simulink model "compareFlexibleCylinders"  (R2023a)
settings: Solver=ode23t  StartTime=0.0  StopTime=2.5  MaxStep=0.01  RelTol=1e-4  AbsTol=1e-5  EnableMultiTasking=on
PreLoadFcn:
  | setup_ROM_validation;
StopFcn:
  | show_SDI_view(ValidationTest)
undefined symbols (not defined in the file): E, L, nu, r, X, Y, Z
libraries: sm_lib x15, nesl_utility x7
settings Model: Creator=dbalbuen  LastModifiedBy=upattacini
settings SolverCC: AutoScaleAbsTol=off  AlgebraicLoopSolver=TrustRegion
settings DataIOCC: MaxDataPoints=10000  SaveOutput=off  DSMLogging=off  SignalLoggingName=logsout_flex_body  DatasetSignalFormat=timetable
settings OptimizationCC: ReuseModelBlockBuffer=off  LifeSpan=inf
settings DebuggingCC: UnconnectedInputMsg=warning  UnconnectedOutputMsg=warning  UnconnectedLineMsg=warning  AllowSymbolicDim=off  SFUnexpectedBacktrackingDiag=warning  SFNoUnconditionalDefaultTransitionDiag=warning  SFExecutionAtInitializationDiag=none  ArithmeticOperatorsInVariantConditions=warning
settings ModelReferenceCC: EnableRefExpFcnMdlSchedulingChecks=on
settings SFSimCC: SimUseLocalCustomCode=off  CustomCodeUndefinedFunction=UseInterfaceOnly
settings RTWCC: RTWUseLocalCustomCode=off  DLArmComputeVersion=19.05
settings CodeAppCC: StateflowObjectComments=on
settings GRTTargetCC: TargetLangStandard=C89/C90 (ANSI)
settings ConfigComp: CovMetricSettings=dw  CovSaveCumulativeToWorkspaceVar=on  CovSaveSingleToWorkspaceVar=on  CovExternalEMLEnable=off  CovSFcnEnable=off
settings SimscapeCC: SimscapeLogType=all  SimscapeLogSimulationStatistics=on  SimscapeLogDataHistory=10000
settings DiagnosticsConfigSet: SimMechanicsInvalidVisualProperty=none
settings ExplorerConfigSet: InternalSimMechanicsExplorerSettings="<ExplorerConfiguration><canonicalview>default</canonicalview><AnimationSetting><BasePlaybackSpeed>1.0</BasePlaybackSpeed><PlaybackSpeedFactor>1.0</PlaybackSpeedFactor></AnimationSetting><TilePanel><TileInfo><Tiles Columns=\"2\" Count=\"2\" Rows=\"1\"><Column Weight=\"0.4996\"/><Column Weight=\"0.5004\"/><Row Weight=\"1\"/><Tile Height=\"1\" Width=\"1\" X=\"0\" Y=\"0\"/><Tile Height=\"1\" Width=\"1\" X=\"1\" Y=\"0\"/></Tiles></TileInfo><SceneInfo><SceneViewer><BGColor><R>1</R><G>1</G><B>1</B></BGColor><Camera><DoPerspective>off</DoPerspective><Position><X>1.10451667165203782</X><Y>-0.556333933861863805</Y><Z>0.510096200126537114</Z></Position><Center><X>0.388367773315445863</X><Y>0.1598149644747279</Y><Z>-0.20605269821005473</Z></Center><Up><X>-0.408248290463863073</X><Y>0.408248290463863073</Y><Z>0.816496580927726145</Z></Up><ViewLimDist>1</ViewLimDist><YLim>0.805305415050960982</YLim><XLim>0.516336295324746897</XLim></Camera></SceneViewer><SceneViewer><BGColor><R>1</R><G>1</G><B>1</B></BGColor><Camera><DoPerspective>off</DoPerspective><Position><X>0.524478029771406673</X><Y>-1.08935703501999259</Y><Z>-0.311817888307719004</Z></Position><Center><X>0.524478029771406673</X><Y>1.33809996694100874e-08</Y><Z>-0.311817888307719004</Z></Center><Up><X>0</X><Y>-0</Y><Z>1</Z></Up><ViewLimDist>1</ViewLimDist><YLim>1.0281975000000001</YLim><XLim>0.660677670375521608</XLim></Camera></SceneViewer></SceneInfo></TilePanel><MechEditorPanel><Cameras/><GfxPanelCameraMap/><VideoCreator><PlaybackSpeedRatio>1.0</PlaybackSpeedRatio><FrameRate>30</FrameRate><VideoFormat>Motion JPEG AVI</VideoFormat><FrameSize>auto</FrameSize></VideoCreator></MechEditorPanel></ExplorerConfiguration>"

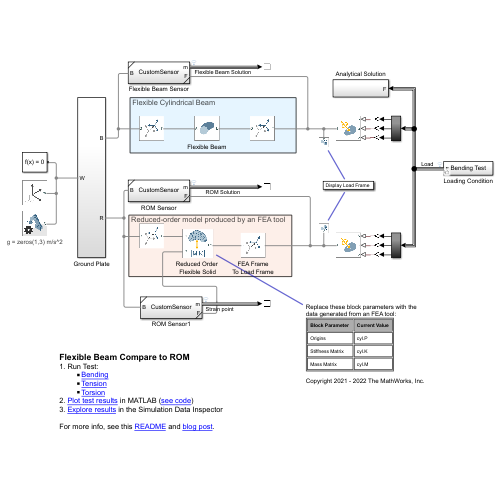
[thumbnail: Simulink's stored preview of the top-level diagram]
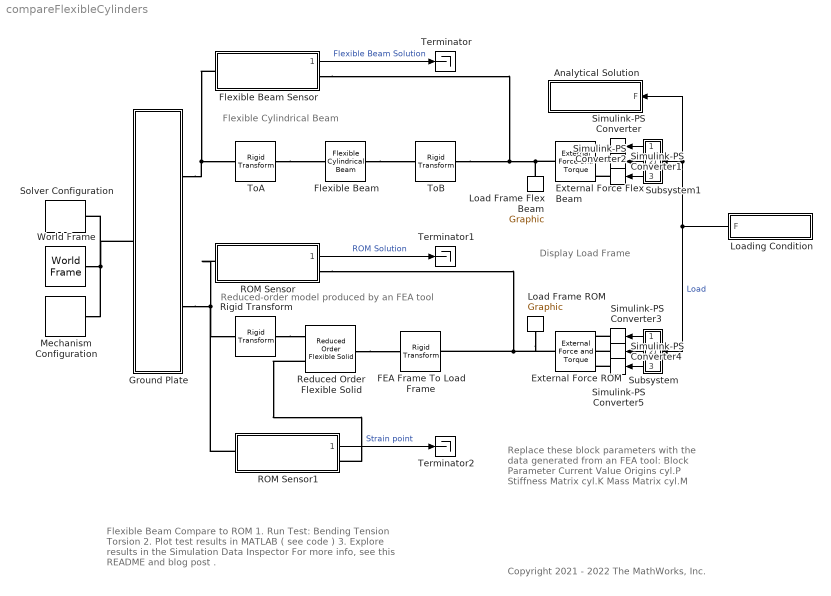
== system compareFlexibleCylinders ==
  note: Display Load Frame
  note: Replace these block parameters with the data generated from an FEA tool:
      |
      | Block Parameter
      | Current Value
      |
      | Origins
      | cyl.P
      |
      | Stiffness Matrix
      | cyl.K
      |
      | Mass Matrix
      | cyl.M
  note: Flexible Cylindrical Beam
  note: Reduced-order model produced by an FEA tool
  note: Flexible Beam Compare to ROM
      | 1. Run Test:
      | Bending
      | Tension
      | Torsion
      | 2. Plot test results in MATLAB ( see code )
      | 3. Explore results in the Simulation Data Inspector
      |
      | For more info, see this README and blog post .
  note: Copyright 2021 - 2022 The MathWorks, Inc.
  Analytical Solution : Subsystem
  External Force Flex Beam : sm_lib/Forces and Torques/External Force and Torque  ForceResolutionFrame=AttachedFrame  EnableForceX=on  EnableForceY=off  EnableForceZ=on  EnableForce=off  TorqueResolutionFrame=AttachedFrame  EnableTorqueX=on  EnableTorqueY=off  EnableTorqueZ=off  EnableTorque=off
  External Force ROM : sm_lib/Forces and Torques/External Force and Torque  ForceResolutionFrame=AttachedFrame  EnableForceX=on  EnableForceY=off  EnableForceZ=on  EnableForce=off  TorqueResolutionFrame=AttachedFrame  EnableTorqueX=on  EnableTorqueY=off  EnableTorqueZ=off  EnableTorque=off
  FEA Frame To Load Frame : sm_lib/Frames and Transforms/Rigid Transform  TranslationMethod=None  TranslationStandardOffset=0  TranslationStandardOffsetUnits=m  TranslationStandardAxis=+Z  TranslationCartesianOffset=[0 0 0]  TranslationCartesianOffsetUnits=m  TranslationROffset=0  TranslationROffsetUnits=m  TranslationZOffset=0  TranslationZOffsetUnits=m  TranslationThetaOffset=0  TranslationThetaOffsetUnits=deg  RotationMethod=StandardAxis  RotationAngleUnits=deg  RotationStandardAxis=+Y  RotationAngle=90  RotationArbitraryAxis=[0 0 1]  FollAlignAxisA=+X  BaseAlignAxisA=+Y  FollAlignAxisB=+Y  BaseAlignAxisB=+Z  RotationSequenceAxes=FollowerAxes  RotationSequence=XYX  RotationSequenceAngles=[0 0 0]  RotationSequenceAnglesUnits=deg  RotationMatrix=[1 0 0; 0 1 0; 0 0 1]  Quaternion=[1 0 0 0]
  Flexible Beam : sm_lib/Body Elements/Flexible Bodies/Beams/Flexible Cylindrical Beam  GraphicAmbientColor=[0.15 0.15 0.15 1.0]  AxialRigidity=1  AxialRigidityUnits=Pa*m^2  BendingCentroid=[0 0]  BendingCentroidUnits=m  FlexuralRigidity=[1 1]  FlexuralRigidityUnits=Pa*m^4  CenterOfMass=[0 0]  CenterOfMassUnits=m  GraphicDiffuseColor=[0.0 0.8 1.0]  CrossFlexuralRigidity=0  CrossFlexuralRigidityUnits=Pa*m^4  SerializedFrames=<Frames/>  DampingType=Proportional  Density=rho  DensityUnits=kg/m^3  DoExposeZmaxFrame=on  DoExposeZminFrame=on  GraphicEmissiveColor=[0.0 0.0 0.0 1.0]  GeometricCentroid=[0 0]  GeometricCentroidUnits=m  GraphicType=FromGeometry  Length=L  LengthUnits=m  MassMomentOfInertiaDensity=[1 1]  MassMomentOfInertiaDensityUnits=kg*m  MassPerUnitLength=1  MassPerUnitLengthUnits=kg/m  MassProductOfInertiaDensity=0  MassProductOfInertiaDensityUnits=kg*m  ModuliType=YoungsPoissons  NumElements=10  NumRetainedModes=1  GraphicOpacity=1  PoissonsRatio=nu  Radius=r  RadiusUnits=m  ReductionType=None  SectionType=Solid  ShearCenter=[0 0]  ShearCenterUnits=m  ShearModulus=26  ShearModulusUnits=GPa  GraphicShininess=75  GraphicSpecularColor=[0.5 0.5 0.5 1.0]  StiffnessAndInertiaType=CalculateFromGeometry  Thickness=0.1  ThicknessUnits=m  TorsionalRigidity=1  TorsionalRigidityUnits=Pa*m^4  GraphicVisPropType=SimpleVisualProperties  YoungsModulus=E  YoungsModulusUnits=Pa  ProportionalDampingAlpha=0  ProportionalDampingAlphaUnits=1/s  ProportionalDampingBeta=Beta  ProportionalDampingBetaUnits=s  UniformModalDampingRatio=0.01
  Flexible Beam Sensor : Subsystem  ReferencedSubsystem=CustomSensor
      settings: PortSchema="{\"entries\":[{\"content\":{\"sides\":[{\"content\":{\"connectorIds\":[\"LConn1\"]},\"type\":\"ConnectorPlacement.EquallySpacedRectSide\",\"uuid\":\"7fafd3ae-1fba-4f09-a97b-f3b2342423e3\"},{\"content\":{\"connectorIds\":[\"RConn1\",\"Out1\"],\"side\":\"RIGHT\"},\"type\":\"ConnectorPlacement.EquallySpacedRectSide\",\"uuid\":\"bc0d00af-c2a5-4688-9bba-52926bbc70a8\"},{\"content\":{\"side\":\"TOP\"},\"type\":\"ConnectorPlacement.EquallySpacedRectSide\",\"uuid\":\"984d0ed5-678d-4848-ae86-c23030322328\"},{\"content\":{\"side\":\"HIDDEN\"},\"type\":\"ConnectorPlacement.EquallySpacedRectSide\",\"uuid\":\"5459c863-0a9c-435c-a481-400fa9a25bf2\"}]},\"type\":\"ConnectorPlacement.EquallySpacedConnector\",\"uuid\":\"ae2cbc6a-d804-41f6-859e-ee34f76c879c\"}],\"packageUris\":[\"http://schema.mathworks.com/mf0/Connector/R2020b\"],\"version\":\"1.0\"}"
  Ground Plate : Subsystem
  Load Frame Flex Beam : sm_lib/Body Elements/Graphic  GraphicType=Marker  MarkerShape=Frame  MarkerSize=30  GraphicVisPropType=SimpleVisualProperties  GraphicDiffuseColor=[0.0 0.0 0.0]  GraphicSpecularColor=[0.5 0.5 0.5 1.0]  GraphicAmbientColor=[0.15 0.15 0.15 1.0]  GraphicEmissiveColor=[0.0 0.0 0.0 1.0]  GraphicShininess=75  GraphicOpacity=1.0
  Load Frame ROM : sm_lib/Body Elements/Graphic  GraphicType=Marker  MarkerShape=Frame  MarkerSize=30  GraphicVisPropType=SimpleVisualProperties  GraphicDiffuseColor=[0.0 0.0 0.0]  GraphicSpecularColor=[0.5 0.5 0.5 1.0]  GraphicAmbientColor=[0.15 0.15 0.15 1.0]  GraphicEmissiveColor=[0.0 0.0 0.0 1.0]  GraphicShininess=75  GraphicOpacity=1.0
  Loading Condition : Subsystem  Variant=on  VariantControl=Choice
  Mechanism Configuration : sm_lib/Utilities/Mechanism Configuration  UniformGravity=Constant  GravityVector=zeros(1,3)  GravityVectorUnits=m/s^2  LinearizationDelta=0.001  JointModeTransitionNonlinearIterations=2
      settings: AttributesFormatString=g = %<GravityVector> %<GravityVectorUnits>
  ROM Sensor : Subsystem  ReferencedSubsystem=CustomSensor
      settings: PortSchema="{\"entries\":[{\"content\":{\"sides\":[{\"content\":{\"connectorIds\":[\"LConn1\"]},\"type\":\"ConnectorPlacement.EquallySpacedRectSide\",\"uuid\":\"7fafd3ae-1fba-4f09-a97b-f3b2342423e3\"},{\"content\":{\"connectorIds\":[\"RConn1\",\"Out1\"],\"side\":\"RIGHT\"},\"type\":\"ConnectorPlacement.EquallySpacedRectSide\",\"uuid\":\"bc0d00af-c2a5-4688-9bba-52926bbc70a8\"},{\"content\":{\"side\":\"TOP\"},\"type\":\"ConnectorPlacement.EquallySpacedRectSide\",\"uuid\":\"984d0ed5-678d-4848-ae86-c23030322328\"},{\"content\":{\"side\":\"HIDDEN\"},\"type\":\"ConnectorPlacement.EquallySpacedRectSide\",\"uuid\":\"5459c863-0a9c-435c-a481-400fa9a25bf2\"}]},\"type\":\"ConnectorPlacement.EquallySpacedConnector\",\"uuid\":\"ae2cbc6a-d804-41f6-859e-ee34f76c879c\"}],\"packageUris\":[\"http://schema.mathworks.com/mf0/Connector/R2020b\"],\"version\":\"1.0\"}"
  ROM Sensor1 : Subsystem  ReferencedSubsystem=CustomSensor
      settings: PortSchema="{\"entries\":[{\"content\":{\"sides\":[{\"content\":{\"connectorIds\":[\"LConn1\"]},\"type\":\"ConnectorPlacement.EquallySpacedRectSide\",\"uuid\":\"7fafd3ae-1fba-4f09-a97b-f3b2342423e3\"},{\"content\":{\"connectorIds\":[\"RConn1\",\"Out1\"],\"side\":\"RIGHT\"},\"type\":\"ConnectorPlacement.EquallySpacedRectSide\",\"uuid\":\"bc0d00af-c2a5-4688-9bba-52926bbc70a8\"},{\"content\":{\"side\":\"TOP\"},\"type\":\"ConnectorPlacement.EquallySpacedRectSide\",\"uuid\":\"984d0ed5-678d-4848-ae86-c23030322328\"},{\"content\":{\"side\":\"HIDDEN\"},\"type\":\"ConnectorPlacement.EquallySpacedRectSide\",\"uuid\":\"5459c863-0a9c-435c-a481-400fa9a25bf2\"}]},\"type\":\"ConnectorPlacement.EquallySpacedConnector\",\"uuid\":\"ae2cbc6a-d804-41f6-859e-ee34f76c879c\"}],\"packageUris\":[\"http://schema.mathworks.com/mf0/Connector/R2020b\"],\"version\":\"1.0\"}"
  Reduced Order Flexible Solid : sm_lib/Body Elements/Flexible Bodies/Reduced Order Flexible Solid  GraphicAmbientColor=[0.15 0.15 0.15 1.0]  GraphicDiffuseColor=[1 0.4118 0.1608]  DampingType=Proportional  GraphicEmissiveColor=[0.0 0.0 0.0 1.0]  GraphicFacetVertexIndices=[]  GeomFileName=Cylinder.stl  InterfaceFrameOrientations=repmat([1 0 0 0],3,1)  GraphicType=PartitionedGeometry  MassMatrix=cyl.M  NumRetainedModes=1  NumberOfInterfaceFrames=3  GraphicOpacity=1.0  GraphicReconstructionMatrix=[]  ReductionType=None  InterfaceFrameOrigins=cyl.P  GraphicShininess=75  GraphicSpecularColor=[0.5 0.5 0.5 1.0]  StiffnessMatrix=cyl.K  GeomUnitType=FromUnitSystem  GraphicVertexCoordinates=[]  VisRecursionLimit=3  GraphicVisPropType=SimpleVisualProperties  LengthUnit=mm  MassUnit=t  TimeUnit=s  UnitSystemType=SI  ProportionalDampingAlpha=0  ProportionalDampingBeta=Beta  UniformModalDampingRatio=0.01  DampingMatrix=[]
  Rigid Transform : sm_lib/Frames and Transforms/Rigid Transform  TranslationMethod=None  TranslationStandardOffset=0  TranslationStandardOffsetUnits=m  TranslationStandardAxis=+Z  TranslationCartesianOffset=[0 0 0]  TranslationCartesianOffsetUnits=m  TranslationROffset=0  TranslationROffsetUnits=m  TranslationZOffset=0  TranslationZOffsetUnits=m  TranslationThetaOffset=0  TranslationThetaOffsetUnits=deg  RotationMethod=StandardAxis  RotationAngleUnits=deg  RotationStandardAxis=+Y  RotationAngle=-90  RotationArbitraryAxis=[0 0 1]  FollAlignAxisA=+X  BaseAlignAxisA=+Y  FollAlignAxisB=+Y  BaseAlignAxisB=+Z  RotationSequenceAxes=FollowerAxes  RotationSequence=XYX  RotationSequenceAngles=[0 0 0]  RotationSequenceAnglesUnits=deg  RotationMatrix=[1 0 0; 0 1 0; 0 0 1]  Quaternion=[1 0 0 0]
  Simulink-PS Converter{,1,3..4} (4 alike) : nesl_utility/Simulink-PS Converter  PhysicalDomain=network_engine_domain  SubClassName=ps_input  LeftPortType=input  RightPortType=output  PseudoPeriodic=off  Frequencies=[]  NoiseDistribution=none  NoiseParameters=[]  Unit=N  AffineConversion=off  FilteringAndDerivatives=provide  SimscapeFilterOrder=1  InputFilterTimeConstant=0.001  UdotUserProvided=0
  Simulink-PS Converter2 : nesl_utility/Simulink-PS Converter  PhysicalDomain=network_engine_domain  SubClassName=ps_input  LeftPortType=input  RightPortType=output  PseudoPeriodic=off  Frequencies=[]  NoiseDistribution=none  NoiseParameters=[]  Unit=N*m  AffineConversion=off  FilteringAndDerivatives=provide  SimscapeFilterOrder=1  InputFilterTimeConstant=0.001  UdotUserProvided=0
  Simulink-PS Converter5 : nesl_utility/Simulink-PS Converter  PhysicalDomain=network_engine_domain  SubClassName=ps_input  LeftPortType=input  RightPortType=output  PseudoPeriodic=off  Frequencies=[]  NoiseDistribution=none  NoiseParameters=[]  Unit=N*m  AffineConversion=off  FilteringAndDerivatives=provide  SimscapeFilterOrder=1  InputFilterTimeConstant=0.001  UdotUserProvided=0
  Solver Configuration : nesl_utility/Solver Configuration  PhysicalDomain=network_engine_domain  SubClassName=solver  LeftPortType=input  RightPortType=generic  Tones=[]  Harmonics=[]  SimulateNoise=off  Profile=off  UseLocalSampling=off  EnableSwitchedLinearOptims=on  FrequencyDomain=off  UseCCode=off  RelTol=0.001  AbsTol=1e-06  MinStep=1e-09  ToWorkspace=off  RevertToSquareIcSolve=off  NumHomotopyIterations=100  PhasorMode=off  PhasorModeNumHarmonics=1  ConsistencySolver=NEWTON_XTOL_AFTER_FTOL  IndexReductionMethod=DerivativeReplacement  DoDC=off  ResidualTolerance=1e-09  ConsistencyTolSource=GLOBAL  ConsistencyAbsTol=0.001  ConsistencyRelTol=0.001  ConsistencyTolFactor=0.001  UseLocalSolver=off  LocalSolverChoice=NE_BACKWARD_EULER_ADVANCER  ResolveIndetEquations=on  FunctionEvalNumThread=1  LocalSolverSampleTime=0.001  DoFixedCost=off  MaxNonlinIter=3  MaxModeIter=2  ComputeImpulses=off  ImpulseIterations=2  LinearAlgebra=Sparse  LinearAlgebraNumThread=0  EquationFormulation=NE_TIME_EF  DelaysMemoryBudget=1024  AutomaticFiltering=on  FilteringTimeConstant=0.001  PartitionStorageMethod=AS_NEEDED  PartitionMemoryBudget=1024  PartitionMethod=FAST
  Subsystem : Subsystem
  Subsystem1 : Subsystem
  Terminator : Terminator
  Terminator1 : Terminator
  Terminator2 : Terminator
  ToA : sm_lib/Frames and Transforms/Rigid Transform  TranslationMethod=None  TranslationStandardOffset=0  TranslationStandardOffsetUnits=m  TranslationStandardAxis=+Z  TranslationCartesianOffset=[0 0 0]  TranslationCartesianOffsetUnits=m  TranslationROffset=0  TranslationROffsetUnits=m  TranslationZOffset=0  TranslationZOffsetUnits=m  TranslationThetaOffset=0  TranslationThetaOffsetUnits=deg  RotationMethod=StandardAxis  RotationAngleUnits=deg  RotationStandardAxis=+Y  RotationAngle=90  RotationArbitraryAxis=[0 0 1]  FollAlignAxisA=+X  BaseAlignAxisA=+Y  FollAlignAxisB=+Y  BaseAlignAxisB=+Z  RotationSequenceAxes=FollowerAxes  RotationSequence=XYX  RotationSequenceAngles=[0 0 0]  RotationSequenceAnglesUnits=deg  RotationMatrix=[1 0 0; 0 1 0; 0 0 1]  Quaternion=[1 0 0 0]
  ToB : sm_lib/Frames and Transforms/Rigid Transform  TranslationMethod=None  TranslationStandardOffset=0  TranslationStandardOffsetUnits=m  TranslationStandardAxis=+Z  TranslationCartesianOffset=[0 0 0]  TranslationCartesianOffsetUnits=m  TranslationROffset=0  TranslationROffsetUnits=m  TranslationZOffset=0  TranslationZOffsetUnits=m  TranslationThetaOffset=0  TranslationThetaOffsetUnits=deg  RotationMethod=StandardAxis  RotationAngleUnits=deg  RotationStandardAxis=+Y  RotationAngle=-90  RotationArbitraryAxis=[0 0 1]  FollAlignAxisA=+X  BaseAlignAxisA=+Y  FollAlignAxisB=+Y  BaseAlignAxisB=+Z  RotationSequenceAxes=FollowerAxes  RotationSequence=XYX  RotationSequenceAngles=[0 0 0]  RotationSequenceAnglesUnits=deg  RotationMatrix=[1 0 0; 0 1 0; 0 0 1]  Quaternion=[1 0 0 0]
  World Frame : sm_lib/Frames and Transforms/World Frame
  wires:
  Flexible Beam Sensor/1 -> Terminator/1  "Flexible Beam Solution"
  ROM Sensor/1 -> Terminator1/1  "ROM Solution"
  Loading Condition/1(F) -> Subsystem1/1(In1), Analytical Solution/1(F), Subsystem/1(In1)  "Load"
  Subsystem/1(<fx>) -> Simulink-PS Converter3/1
  Subsystem/2(<fz>) -> Simulink-PS Converter4/1
  Subsystem/3(<tx>) -> Simulink-PS Converter5/1
  Subsystem1/1(<fx>) -> Simulink-PS Converter/1
  Subsystem1/2(<fz>) -> Simulink-PS Converter1/1
  Subsystem1/3(<tx>) -> Simulink-PS Converter2/1
  ROM Sensor1/1 -> Terminator2/1  "Strain point"
  connections:
  ROM Sensor/LConn1 -- ROM Sensor1/LConn1 -- Rigid Transform/LConn1 -- Ground Plate/RConn2
  Flexible Beam Sensor/RConn1 -- External Force Flex Beam/RConn1 -- Load Frame Flex Beam/RConn1 -- ToB/RConn1
  Rigid Transform/RConn1 -- Reduced Order Flexible Solid/LConn1
  External Force ROM/RConn1 -- Load Frame ROM/RConn1 -- ROM Sensor/RConn1 -- FEA Frame To Load Frame/RConn1
  Reduced Order Flexible Solid/RConn1 -- FEA Frame To Load Frame/LConn1
  Flexible Beam Sensor/LConn1 -- Ground Plate/RConn1 -- ToA/LConn1
  ToA/RConn1 -- Flexible Beam/LConn1
  Flexible Beam/RConn1 -- ToB/LConn1
  Mechanism Configuration/RConn1 -- Solver Configuration/RConn1 -- Ground Plate/LConn1 -- World Frame/RConn1
  Simulink-PS Converter1/RConn1 -- External Force Flex Beam/LConn2
  Simulink-PS Converter4/RConn1 -- External Force ROM/LConn2
  Simulink-PS Converter2/RConn1 -- External Force Flex Beam/LConn3
  Simulink-PS Converter5/RConn1 -- External Force ROM/LConn3
  Simulink-PS Converter/RConn1 -- External Force Flex Beam/LConn1
  Simulink-PS Converter3/RConn1 -- External Force ROM/LConn1
  Reduced Order Flexible Solid/LConn2 -- ROM Sensor1/RConn1

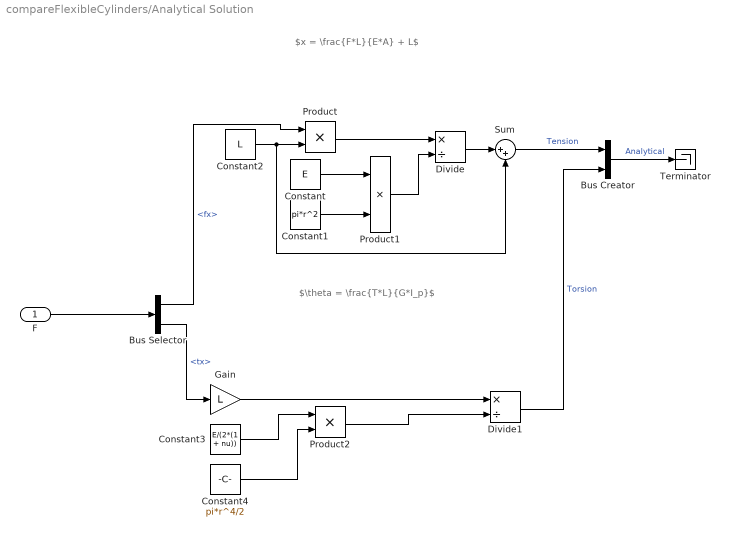
== system compareFlexibleCylinders/Analytical Solution ==
  note: $x = \frac{F*L}{E*A} + L$
  note: $\theta = \frac{T*L}{G*I_p}$
  F : Inport
  Bus Creator : BusCreator  Inputs=2
  Bus Selector : BusSelector  OutputSignals=fx,tx
  Constant : Constant  Value=E
  Constant1 : Constant  Value=pi*r^2
  Constant2 : Constant  Value=L
  Constant3 : Constant  Value=E/(2*(1 + nu))
  Constant4 : Constant  Value=pi*r^4/2
  Divide : Product  Inputs=*/
  Divide1 : Product  Inputs=*/
  Gain : Gain  Gain=L
  Product : Product
  Product1 : Product
  Product2 : Product
  Sum : Sum  Inputs=|++
  Terminator : Terminator
  wires:
  Sum/1 -> Bus Creator/1  "Tension"
  Divide/1 -> Sum/1
  Product1/1 -> Divide/2
  Product/1 -> Divide/1
  Constant/1 -> Product1/1
  Constant1/1 -> Product1/2
  Constant2/1 -> Product/2, Sum/2
  Bus Selector/2 -> Gain/1  "<tx>"
  Constant3/1 -> Product2/1
  Gain/1 -> Divide1/1
  Constant4/1 -> Product2/2
  Divide1/1 -> Bus Creator/2  "Torsion"
  Product2/1 -> Divide1/2
  F/1 -> Bus Selector/1
  Bus Creator/1 -> Terminator/1  "Analytical"
  Bus Selector/1 -> Product/1  "<fx>"

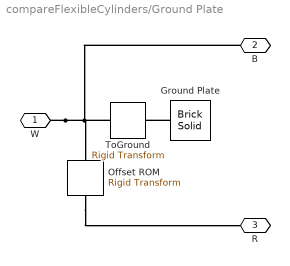
== system compareFlexibleCylinders/Ground Plate ==
  Ground Plate : sm_lib/Body Elements/Brick Solid  GraphicAmbientColor=[0.15 0.15 0.15 1.0]  BasedOnType=Mass  BrickDimensions=[0.01 0.2 1.5]  BrickDimensionsUnits=m  CenterOfMass=[0 0 0]  CenterOfMassUnits=m  GraphicDiffuseColor=[0.8 0.8 0.8]  Density=1000  DensityUnits=kg/m^3  DoExposeReferenceFrame=on  GraphicEmissiveColor=[0.0 0.0 0.0 1.0]  ExportEntireGeometry=off  SerializedFrames=<Frames/>  MarkerShape=Sphere  MarkerSize=10  GraphicType=FromGeometry  InertiaType=PointMass  Mass=0  MassUnits=kg  MomentsOfInertia=[1 1 1]  MomentsOfInertiaUnits=kg*m^2  GraphicOpacity=1  ProductsOfInertia=[0 0 0]  ProductsOfInertiaUnits=kg*m^2  GraphicShininess=75  GraphicSpecularColor=[0.5 0.5 0.5 1.0]  GraphicVisPropType=SimpleVisualProperties
  Offset ROM : sm_lib/Frames and Transforms/Rigid Transform  TranslationMethod=StandardAxis  TranslationStandardOffset=-0.4  TranslationStandardOffsetUnits=m  TranslationStandardAxis=+Z  TranslationCartesianOffset=[0 0 0]  TranslationCartesianOffsetUnits=m  TranslationROffset=0  TranslationROffsetUnits=m  TranslationZOffset=0  TranslationZOffsetUnits=m  TranslationThetaOffset=0  TranslationThetaOffsetUnits=deg  RotationMethod=None  RotationAngleUnits=deg  RotationStandardAxis=+Z  RotationAngle=0.0  RotationArbitraryAxis=[0 0 1]  FollAlignAxisA=+X  BaseAlignAxisA=+Y  FollAlignAxisB=+Y  BaseAlignAxisB=+Z  RotationSequenceAxes=FollowerAxes  RotationSequence=XYX  RotationSequenceAngles=[0 0 0]  RotationSequenceAnglesUnits=deg  RotationMatrix=[1 0 0; 0 1 0; 0 0 1]  Quaternion=[1 0 0 0]
  ToGround : sm_lib/Frames and Transforms/Rigid Transform  TranslationMethod=StandardAxis  TranslationStandardOffset=0.2  TranslationStandardOffsetUnits=m  TranslationStandardAxis=+Z  TranslationCartesianOffset=[0 0 0]  TranslationCartesianOffsetUnits=m  TranslationROffset=0  TranslationROffsetUnits=m  TranslationZOffset=0  TranslationZOffsetUnits=m  TranslationThetaOffset=0  TranslationThetaOffsetUnits=deg  RotationMethod=None  RotationAngleUnits=deg  RotationStandardAxis=+Z  RotationAngle=0.0  RotationArbitraryAxis=[0 0 1]  FollAlignAxisA=+X  BaseAlignAxisA=+Y  FollAlignAxisB=+Y  BaseAlignAxisB=+Z  RotationSequenceAxes=FollowerAxes  RotationSequence=XYX  RotationSequenceAngles=[0 0 0]  RotationSequenceAnglesUnits=deg  RotationMatrix=[1 0 0; 0 1 0; 0 0 1]  Quaternion=[1 0 0 0]
  W : PMIOPort  Side=Left
  B : PMIOPort  Port=2  Side=Right
  R : PMIOPort  Port=3  Side=Right
  connections:
  Offset ROM/RConn1 -- R/RConn1
  Ground Plate/RConn1 -- ToGround/LConn1
  W/RConn1 -- ToGround/RConn1 -- Offset ROM/LConn1 -- B/RConn1

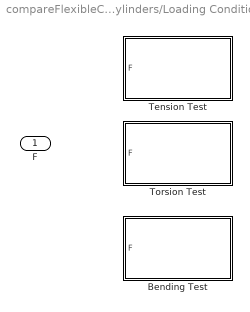
== system compareFlexibleCylinders/Loading Condition ==
  Bending Test : Subsystem  VariantControl=ValidationTest == ValidationType.BENDING
  Tension Test : Subsystem  VariantControl=ValidationTest == ValidationType.TENSION
  Torsion Test : Subsystem  VariantControl=ValidationTest == ValidationType.TORSION
  F : Outport

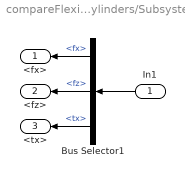
== system compareFlexibleCylinders/Subsystem ==
  In1 : Inport
  Bus Selector1 : BusSelector  OutputSignals=fx,fz,tx
  <fx> : Outport
  <fz> : Outport  Port=2
  <tx> : Outport  Port=3
  wires:
  Bus Selector1/2 -> <fz>/1  "<fz>"
  Bus Selector1/3 -> <tx>/1  "<tx>"
  Bus Selector1/1 -> <fx>/1  "<fx>"
  In1/1 -> Bus Selector1/1

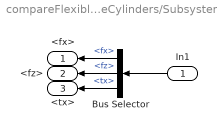
== system compareFlexibleCylinders/Subsystem1 ==
  In1 : Inport
  Bus Selector : BusSelector  OutputSignals=fx,fz,tx
  <fx> : Outport
  <fz> : Outport  Port=2
  <tx> : Outport  Port=3
  wires:
  Bus Selector/3 -> <tx>/1  "<tx>"
  In1/1 -> Bus Selector/1
  Bus Selector/1 -> <fx>/1  "<fx>"
  Bus Selector/2 -> <fz>/1  "<fz>"

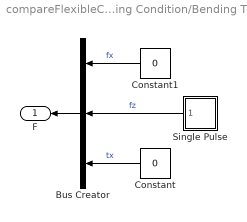
== system compareFlexibleCylinders/Loading Condition/Bending Test ==
  Bus Creator : BusCreator  Inputs=3
  Constant : Constant  Value=0
  Constant1 : Constant  Value=0
  Single Pulse : Subsystem  TreatAsAtomicUnit=on  SystemSampleTime=0  mask{force_mag=1e4}
      mask prompts: force_mag "Force Magnitude"
  F : Outport
  wires:
  Bus Creator/1 -> F/1
  Constant/1 -> Bus Creator/3  "tx"
  Constant1/1 -> Bus Creator/1  "fx"
  Single Pulse/1(Out1) -> Bus Creator/2  "fz"

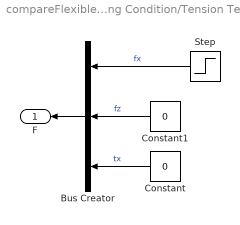
== system compareFlexibleCylinders/Loading Condition/Tension Test ==
  Bus Creator : BusCreator  Inputs=3
  Constant : Constant  Value=0
  Constant1 : Constant  Value=0
  Step : Step  After=10000  SampleTime=0
  F : Outport
  wires:
  Constant/1 -> Bus Creator/3  "tx"
  Constant1/1 -> Bus Creator/2  "fz"
  Step/1 -> Bus Creator/1  "fx"
  Bus Creator/1 -> F/1

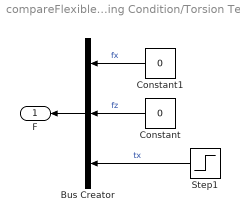
== system compareFlexibleCylinders/Loading Condition/Torsion Test ==
  Bus Creator : BusCreator  Inputs=3
  Constant : Constant  Value=0
  Constant1 : Constant  Value=0
  Step1 : Step  After=1e4  SampleTime=0
  F : Outport
  wires:
  Bus Creator/1 -> F/1
  Step1/1 -> Bus Creator/3  "tx"
  Constant1/1 -> Bus Creator/1  "fx"
  Constant/1 -> Bus Creator/2  "fz"

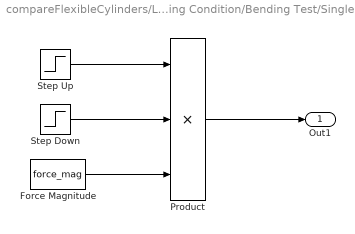
== system compareFlexibleCylinders/Loading Condition/Bending Test/Single Pulse ==
  Force Magnitude : Constant  Value=force_mag
  Product : Product  Inputs=3
  Step Down : Step  Time=1.5  Before=1  After=0  SampleTime=0
  Step Up : Step  SampleTime=0
  Out1 : Outport
  wires:
  Product/1 -> Out1/1
  Force Magnitude/1 -> Product/3
  Step Down/1 -> Product/2
  Step Up/1 -> Product/1
